simulink model "Hochhaus_Simulink"  (R2019b)
settings: Solver=FixedStepAuto  StartTime=0  StopTime=6  FixedStep=0.0005  MaxStep=0.0015  RelTol=1e-3
values from neighbouring files (symbols this model uses):
  fs = 2e3    (= 2000)    [Sim_Plot.m]
undefined symbols (not defined in the file or in its folder): ssmodal
settings Model: Creator=huelsebrock  LastModifiedBy=cy511
settings SFSimCC: CustomCodeUndefinedFunction=UseInterfaceOnly

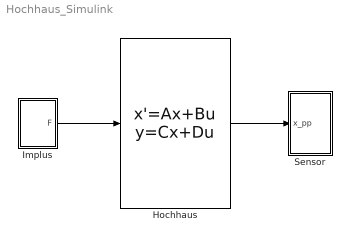
== system Hochhaus_Simulink ==
  Hochhaus : StateSpace  A=ssmodal.a  B=ssmodal.b  C=ssmodal.c  D=ssmodal.d  InitialCondition=0
  Implus : Subsystem
  Sensor : Subsystem
  wires:
  Hochhaus/1 -> Sensor/1(x_pp)
  Implus/1(F) -> Hochhaus/1

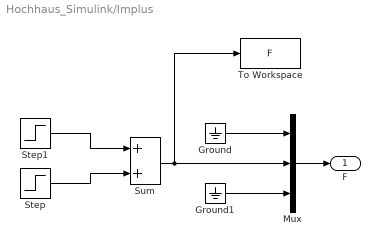
== system Hochhaus_Simulink/Implus ==
  Ground : Ground
  Ground1 : Ground
  Mux : Mux  Inputs=3
  Step : Step  Time=2/fs  After=-1/fs  SampleTime=0
  Step1 : Step  Time=1/fs  After=1/fs  SampleTime=0
  Sum : Sum
  To Workspace : ToWorkspace  VariableName=F  SaveFormat=Timeseries  SampleTime=-1
  F : Outport  VectorParamsAs1DForOutWhenUnconnected=off
  wires:
  Step/1 -> Sum/2
  Step1/1 -> Sum/1
  Mux/1 -> F/1
  Ground/1 -> Mux/1
  Ground1/1 -> Mux/3
  Sum/1 -> Mux/2, To Workspace/1

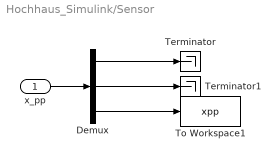
== system Hochhaus_Simulink/Sensor ==
  x_pp : Inport
  Demux : Demux  Outputs=3
  Terminator : Terminator
  Terminator1 : Terminator
  To Workspace1 : ToWorkspace  VariableName=xpp  SampleTime=-1
      settings: Save2DSignal=2-D array (concatenate along first dimension)
  wires:
  x_pp/1 -> Demux/1
  Demux/3 -> To Workspace1/1
  Demux/2 -> Terminator1/1
  Demux/1 -> Terminator/1
